simulink model "Dead_Zone_verif"  (Simulink 8.4)
settings: Solver=ode45  StartTime=0.0  StopTime=10.0  RelTol=1e-3
undefined symbols (not defined in the file): sigbuilder_block
settings Model: Creator=Romain  LastModifiedBy=hbourbou
settings DataIOCC: SignalLoggingSaveFormat=Dataset
settings OptimizationCC: ExpressionDepthLimit=128
settings DebuggingCC: SolverPrmCheckMsg=none  FcnCallInpInsideContextMsg=EnableAllAsError  FrameProcessingCompatibilityMsg=error  StateNameClashWarn=none
settings GRTTargetCC: CombineOutputUpdateFcns=on  GRTInterface=off

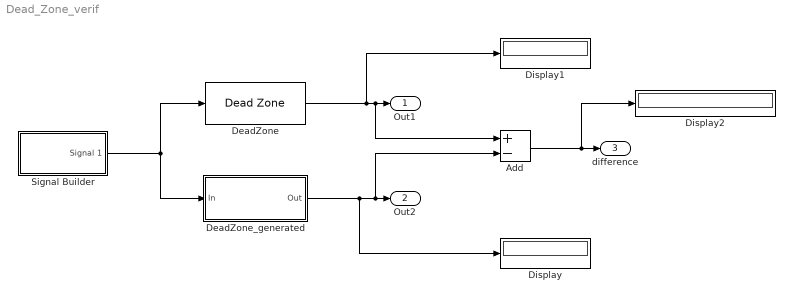
== system Dead_Zone_verif ==
  Add : Sum  Inputs=+-
  DeadZone : DeadZone  SaturateOnIntegerOverflow=on
  DeadZone_generated : Subsystem  TreatAsAtomicUnit=on
  Display : Display
  Display1 : Display
  Display2 : Display
  Signal Builder : Subsystem  Tag=STV Subsys  LoadFcn=sigbuilder_block('load');  StartFcn=sigbuilder_block('start');  StopFcn=sigbuilder_block('stop');  ClipboardFcn=sigbuilder_block('clipboard');  mask(Sigbuilder block){}
      mask help: Simulink:masks:SigbuilderBlock_MD
      mask init:
      | if ~strcmp(get_param(bdroot(gcbh),'SimulationStatus'),'stopped') tuvar = sigbuilder_block('maskInit'); end
      settings: CopyFcn=sigbuilder_block('copy');  DeleteFcn=sigbuilder_block('delete');  ModelCloseFcn=sigbuilder_block('modelClose');  PreSaveFcn=sigbuilder_block('preSave');  PauseFcn=sigbuilder_block('pause');  ContinueFcn=sigbuilder_block('continue');  NameChangeFcn=sigbuilder_block('namechange');  OpenFcn=sigbuilder_block('open',[437.6 199.2 550.4 400 ]);  CloseFcn=sigbuilder_block('close');
      mask Display: plot(0, 0, 100, 100,[2, 2, 32, 32, 2], [68, 8, 8, 68, 68],[32, 2], [38, 38], [32, 19, 2],[53, 60, 44], [32, 17, 17, 2],[16, 16, 31, 31]);txt = getActiveGroup(gcbh);text(2, 100, txt,'verticalAlignment', 'top');
  Out1 : Outport
  Out2 : Outport  Port=2
  difference : Outport  Port=3
  wires:
  Signal Builder/1(Signal 1) -> DeadZone_generated/1(In), DeadZone/1
  DeadZone/1 -> Display1/1, Add/1, Out1/1
  DeadZone_generated/1(Out) -> Display/1, Add/2, Out2/1
  Add/1 -> Display2/1, difference/1

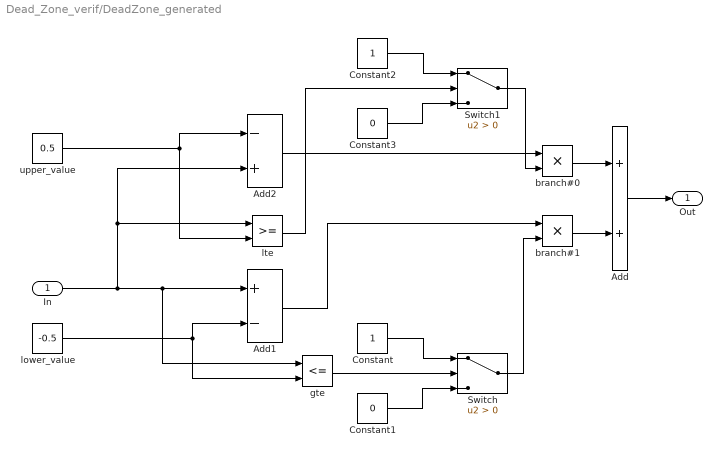
== system Dead_Zone_verif/DeadZone_generated ==
  In : Inport
  Add : Sum
  Add1 : Sum  Inputs=+-
  Add2 : Sum  Inputs=-+
  Constant : Constant
  Constant1 : Constant  Value=0
  Constant2 : Constant
  Constant3 : Constant  Value=0
  Switch : Switch  Criteria=u2 > Threshold
  Switch1 : Switch  Criteria=u2 > Threshold
  branch#0 : Product  RndMeth=Zero
  branch#1 : Product  RndMeth=Zero
  gte : RelationalOperator  Operator=<=  OutDataTypeStr=boolean
  lower_value : Constant  Value=-0.5  SampleTime=-1
  lte : RelationalOperator  OutDataTypeStr=boolean
  upper_value : Constant  Value=0.5  SampleTime=-1
  Out : Outport
  wires:
  In/1 -> Add1/1, gte/1, Add2/2, lte/1
  lower_value/1 -> Add1/2, gte/2
  Add/1 -> Out/1
  upper_value/1 -> Add2/1, lte/2
  Add2/1 -> branch#0/1
  branch#0/1 -> Add/1
  Add1/1 -> branch#1/1
  gte/1 -> Switch/2
  branch#1/1 -> Add/2
  Constant/1 -> Switch/1
  Constant1/1 -> Switch/3
  Switch/1 -> branch#1/2
  lte/1 -> Switch1/2
  Constant2/1 -> Switch1/1
  Constant3/1 -> Switch1/3
  Switch1/1 -> branch#0/2

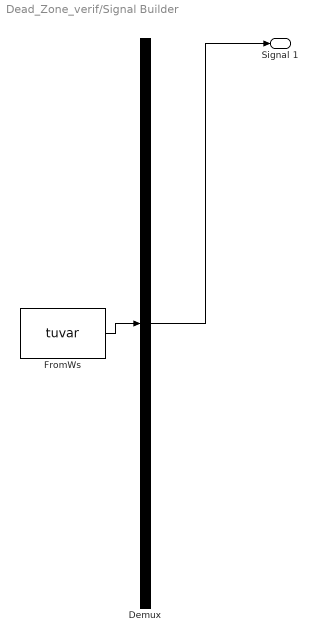
== system Dead_Zone_verif/Signal Builder ==
  Demux : Demux  Tag=STV Demux  Outputs=1
  FromWs : FromWorkspace  Tag=STV FromWs  VariableName=tuvar  SampleTime=0  SigBuilderData=DataTag0  VnvData=DataTag1
      SigBuilderData=|
      | common.afterFinalStr = 'Extrapolate'
      | common.sampleTime = 0
      | dataSet.timeRange = [0 10]
      | dataSet.name = 'Group 1'
      | sbobj.Groups.Name = 'Group 1'
      | sbobj.Groups.Signals.Name = 'Signal 1'
      | sbobj.Groups.Signals.XData = [0 4 4 6 6 10]
      | sbobj.Groups.Signals.YData = [0 0.99 1 0.3 0.26 0]
  Signal 1 : Outport  Tag=STV Outport
  wires:
  Demux/1 -> Signal 1/1
  FromWs/1 -> Demux/1
